simulink model "exampleLoopSimscape"  (R2024b)
settings: Solver=VariableStepAuto  StartTime=0.0  StopTime=10.0  RelTol=1e-3
settings Model: Creator=grouleau  LastModifiedBy=grouleau
settings ModelReferenceCC: UpdateModelReferenceTargets=IfOutOfDate  ModelReferenceMinAlgLoopOccurrences=on

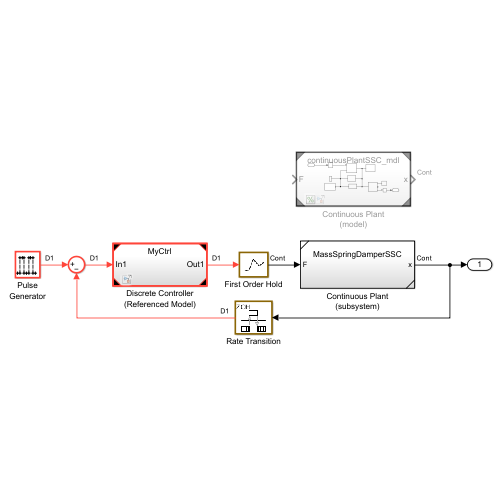
[thumbnail: Simulink's stored preview of the top-level diagram]
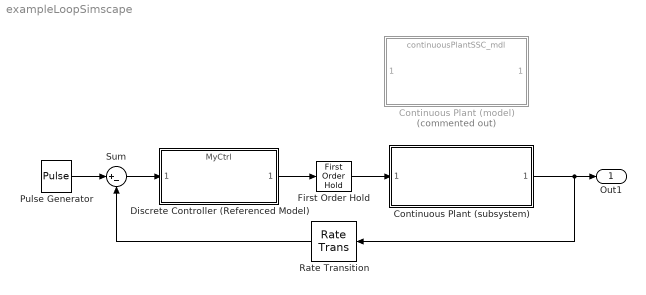
== system exampleLoopSimscape ==
  Continuous Plant (model) : ModelReference  Commented=on  ModelNameDialog=continuousPlantSSC_mdl.slx  ModelReferenceVersion=1.3
  Continuous Plant (subsystem) : Subsystem  ReferencedSubsystem=MassSpringDamperSSC
  Discrete Controller (Referenced Model) : ModelReference  ModelNameDialog=MyCtrl  ModelReferenceVersion=1.6
  First Order Hold : FirstOrderHold  ErrorTolerance=inf
  Pulse Generator : DiscretePulseGenerator  Period=4000  PulseWidth=2000  SampleTime=0.001
  Rate Transition : RateTransition  OutPortSampleTime=0.001
  Sum : Sum  Inputs=|+-
  Out1 : Outport
  wires:
  Pulse Generator/1 -> Sum/1
  Sum/1 -> Discrete Controller (Referenced Model)/1
  Discrete Controller (Referenced Model)/1 -> First Order Hold/1
  First Order Hold/1 -> Continuous Plant (subsystem)/1
  Continuous Plant (subsystem)/1 -> Rate Transition/1, Out1/1
  Rate Transition/1 -> Sum/2
